simulink model "Stateflow_action2"  (R2016b)
settings: Solver=VariableStepAuto  StartTime=0.0  StopTime=10.0  RelTol=1e-3  EnableMultiTasking=on
settings Model: Creator=amyyang  LastModifiedBy=amyyang
settings DataIOCC: LimitDataPoints=on
settings OptimizationCC: LifeSpan=inf
settings DebuggingCC: AllowSymbolicDim=off  SFUnexpectedBacktrackingDiag=warning  SFNoUnconditionalDefaultTransitionDiag=warning  SFExecutionAtInitializationDiag=none
settings ModelReferenceCC: PropagateSignalLabelsOutOfModel=off
settings GRTTargetCC: TargetLangStandard=C89/C90 (ANSI)
settings ConfigComp: CovMetricSettings=dw  CovHtmlReporting=on  CovSaveCumulativeToWorkspaceVar=on  CovSaveSingleToWorkspaceVar=on  CovExternalEMLEnable=off

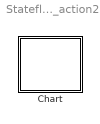
== system Stateflow_action2 ==
  Chart : Stateflow chart  TreatAsAtomicUnit=on

== stateflow chart Stateflow_action2/Chart ==
  state Correct10 [parallel]
    settings: executionOrder=1
  state InCorrect11 [parallel]
    settings: executionOrder=2
  note: 最好不要使用
      | transition Action
  state ? [parallel]
    settings: executionOrder=3
  state ? [parallel]
    settings: executionOrder=4
  state A [parallel]
    settings: executionOrder=5
    state Correct11
    state C
    (default) -> Correct11
    Correct11 -> (junction 155) : [ Condition1]
        | {
        |  Action1;
        | }
    (junction 155) -> A.C : {
        |  conditonaction;
        | }
  state B [parallel]
    settings: executionOrder=6
    state InCorrect12
    state C2
    (default) -> InCorrect12
    InCorrect12 -> (junction 151) : [ Condition1]
        | {
        | Action1;
        | }
    (junction 151) -> C2 : /{ transitionAction;}
  note: 一定不要混用
      | transition Action
      | 和conditon action
  state C [parallel]
    settings: executionOrder=7
    state AA
    state AB
    (default) -> C.AA
    C.AA -> C.AB : /{action1;action2;}
  state C1 [parallel]
    settings: executionOrder=8
    state AA
    state AB
    (default) -> C1.AA
    C1.AA -> C1.AB : /{action1;}
  Correct10 -> ? : [ Condition1]
      | {
      |  Action1;
      | }
  InCorrect11 -> ? : [ Condition1]
      | /  transitionAction;
